simulink model "solution_ImageClassification"  (R2023a)
settings: Solver=VariableStepAuto  StartTime=0.0  StopTime=10.0  RelTol=1e-3
libraries: deeplib x1, visionsources x1
settings Model: Creator=gracew  LastModifiedBy=gracew
settings OptimizationCC: ReuseModelBlockBuffer=off

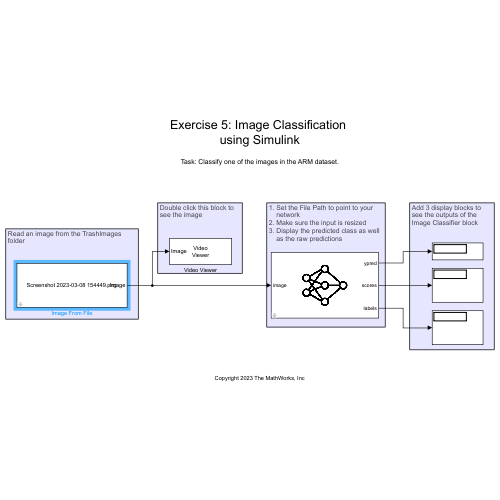
[thumbnail: Simulink's stored preview of the top-level diagram]
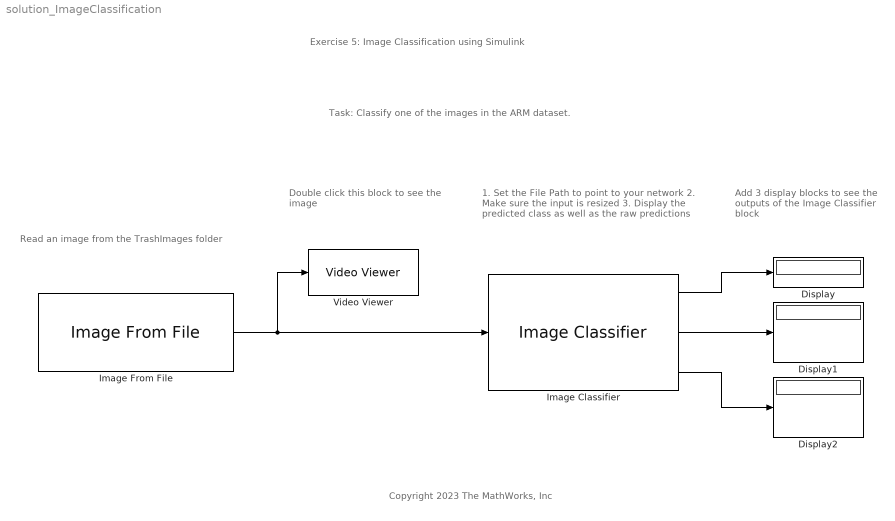
== system solution_ImageClassification ==
  note: Copyright 2023 The MathWorks, Inc
  note: Add 3 display blocks to
      | see the outputs of the
      | Image Classifier block
  note: Double click this block to
      | see the image
  note: 1. Set the File Path to point to your
      |     network
      | 2. Make sure the input is resized
      | 3. Display the predicted class as well
      |     as the raw predictions
  note: Read an image from the TrashImages
      | folder
  note: Task: Classify one of the images in the ARM dataset.
  note: Exercise 5: Image Classification
      | using Simulink
  Display : Display
  Display1 : Display
  Display2 : Display
  Image Classifier : deeplib/Image Classifier  Network=Network from MAT-file  NetworkFunction=squeezenet  NetworkFilePath=C:\Users\gracew\OneDrive - MathWorks\_MyFolders\Engagements\Making Vehicles and Robots See\Image Classification\mynet.mat  MiniBatchSize=128  ResizeInput=on  Classification=on  Predictions=on  ForceInterpretedSim=off  PredictMode=All probabilities and labels  K=5
  Image From File : visionsources/Image From File  Tag=vipblks_nd  FileName=C:\Users\gracew\OneDrive - MathWorks\_MyFolders\Engagements\Making Vehicles and Robots See\Image Classification\ARMImages\detergent\Screenshot 2023-03-08 154449.png  Ts=inf  imagePorts=One multidimensional signal  OutPortLabels=R|G|B  ImageDataType=Inherit from input image  sdImageDataType=uint(8)  Signed=on  WordLength=16  FractionLengthMode=User-defined  FractionLength=15
  Video Viewer : VideoViewer  FigPos=[2041 741 418 304]
  wires:
  Image From File/1 -> Video Viewer/1, Image Classifier/1
  Image Classifier/1 -> Display/1
  Image Classifier/2 -> Display1/1
  Image Classifier/3 -> Display2/1
